simulink model "ecualizador"  (R2017a)
settings: Solver=FixedStepDiscrete  StartTime=0.0  StopTime=Inf  RelTol=1e-3  EnableMultiTasking=on
libraries: dsparch4 x7, dspsrcs4 x3, dspvision x1
settings Model: Creator=The MathWorks, Inc.  LastModifiedBy=hmartiney
settings DataIOCC: LimitDataPoints=on  SaveFormat=Array
settings OptimizationCC: LifeSpan=inf
settings DebuggingCC: SolverPrmCheckMsg=warning  AllowSymbolicDim=off  SFUnexpectedBacktrackingDiag=warning  SFNoUnconditionalDefaultTransitionDiag=warning  SFExecutionAtInitializationDiag=none
settings HardwareCC: ProdBitPerPointer=32  ProdBitPerSizeT=32  ProdBitPerPtrDiffT=32  ProdLargestAtomicFloat=None  ProdIntDivRoundTo=Undefined  ProdEndianess=Unspecified  ProdWordSize=32  ProdHWDeviceType=32-bit Generic
settings ModelReferenceCC: PropagateSignalLabelsOutOfModel=off
settings GRTTargetCC: TargetLangStandard=C89/C90 (ANSI)  GeneratePreprocessorConditionals=Disable all
settings ConfigComp: CovMetricSettings=dw  CovHtmlReporting=on  CovSaveCumulativeToWorkspaceVar=on  CovSaveSingleToWorkspaceVar=on  CovExternalEMLEnable=off  CovSFcnEnable=off

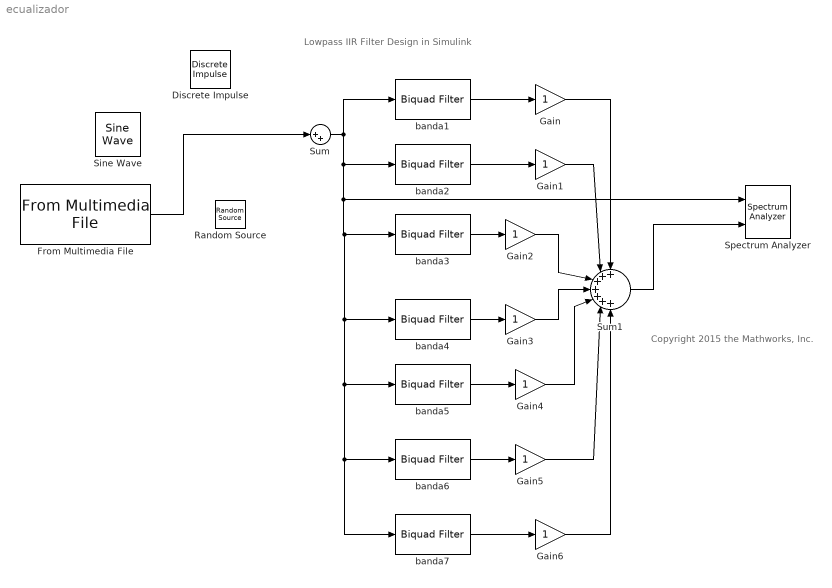
== system ecualizador ==
  note: Copyright 2015 the Mathworks, Inc.
  note: Lowpass IIR Filter Design in Simulink
  Discrete Impulse : dspsrcs4/Discrete  Impulse  Delay=0  SampleTime=1  FrameSample=1  OutputFrames=off  dataType=double  isSigned=on  wordLen=16  udDataType=sfix(16)  fracBitsMode=Best precision  numFracBits=15  OutDataTypeStr=double  LastOutDataTypeStr=double
  From Multimedia File : dspvision/From Multimedia File  inputFilename=/Users/hmartiney/DSPEqualizerProject/1-01 Out My Head (www.hiphopeasy.com).mp3  loop=on  numPlays=inf  outputStreams=Audio only  videoDataType=single  audioDataType=double  inheritSampleTime=on  userDefinedSampleTime=1/30  noAudioOutput=off  isIntensityVideo=off  fourcc=RGB  colorVideoFormat=Separate color signals  outputEOF=off  dataOrg=Column-major  audioFrameSize=1024  computeAudioFrameSize=off  outSamplingMode=Sample based
      settings: SourceProductBaseCode=VP
  Gain{,1..6} (7 alike) : Gain
  Random Source : dspsrcs4/Random Source  SrcType=Gaussian  NormMethod=Ziggurat  CltLength=12  MinVal=0  MaxVal=1  MeanVal=0  VarVal=1e-5  RepMode=Specify seed  rawSeed=1  IsInherit=off  SampMode=Discrete  SampTime=1/44100  SampFrame=1024  DataType=Double  OutComplex=Real  OutputFrames=off
  Sine Wave : dspsrcs4/Sine Wave  Amplitude=1  Frequency=100  Phase=0  SampleMode=Discrete  OutComplex=Real  CompMethod=Trigonometric fcn  TableSize=Speed  SampleTime=1/44100  SamplesPerFrame=1024  ResetState=Restart at time zero  OutputFrames=off  dataType=double  wordLen=16  udDataType=sfix(16)  fracBitsMode=Best precision  numFracBits=15  OutDataTypeStr=double  LastOutDataTypeStr=double
  Spectrum Analyzer : SpectrumAnalyzer  NumInputPorts=2
  Sum : Sum  Inputs=|++
  Sum1 : Sum  Inputs=+++++++
  banda1 : dsparch4/Biquad Filter  Tag=BlockMethodSubSystem  IIRFiltStruct=Direct form II  CoeffSource=Specify via dialog  BiQuadCoeffs=[0.00018458300227112165 -0.00036906768600448764 0.000184583002271121677 1 -1.99947854026079197 0.999478638598126135;0.00057538077100641725 -0.00115066319336694063 0.000575380771006417358 1 -1.99987759640344676 0.9998776947219844;2.27833399804225939e-05 -4.54683566244835644e-05 2.27833399804225905e-05 1 -1.99938484320312182 0.999384941551767825;1.00011892756945397 -2 1.00011892756945375 1 -1.99965158871292981 0.999651687036266057]  a0Flag=Warning  IC=0  ICnum=0  ICden=0  InputProcessing=Columns as channels (frame based)  denAccumFracLength=30  denProdOutputFracLength=30  secondMemoryFracLength=15  roundingMode=Floor  overflowMode=off  ScaleValues=[9.83373342755555768e-08;1;1;1;4204.23962093165483]  optimizeScaleValues=on  ScaleValueMode=Specify via input port (g)  scaleValueFracLength=14  FilterSource=Specify via dialog  FilterObject=BQF
      settings: SourceProductName=DSP System Toolbox
  banda2 : dsparch4/Biquad Filter  Tag=BlockMethodSubSystem  IIRFiltStruct=Direct form II  CoeffSource=Specify via dialog  BiQuadCoeffs=[0.192137146734570385 -0.384037148070295542 0.192137146734570385 1 -1.99777092121242461 0.999494811108345704;0.0756226935951563178 -0.151052150183008216 0.075622693595156304 1 -1.99765102526638483 0.999479693593270158;0.0721798852515740386 -0.144305358912791171 0.0721798852515740663 1 -1.99700920616910249 0.998762370564236002;1.00209566000222439 -1.99999999999999978 1.00209566000222439 1 -1.99695025262914783 0.99874706897447596]  a0Flag=Warning  IC=0  ICnum=0  ICden=0  InputProcessing=Columns as channels (frame based)  denAccumFracLength=30  denProdOutputFracLength=30  secondMemoryFracLength=15  roundingMode=Floor  overflowMode=off  ScaleValues=[2.28356136424982117e-05;1;1;1;416.112600169732445]  optimizeScaleValues=on  ScaleValueMode=Specify via input port (g)  scaleValueFracLength=14  FilterSource=Specify via dialog  FilterObject=BQF
      settings: SourceProductName=DSP System Toolbox
  banda3 : dsparch4/Biquad Filter  Tag=BlockMethodSubSystem  IIRFiltStruct=Direct form II  CoeffSource=Specify via dialog  BiQuadCoeffs=[0.180047662333926051 -0.359206709516307732 0.180047662333926051 1 -1.99209861256290632 0.998989800786029836;0.0769354203253417995 -0.153084985509638283 0.0769354203253417857 1 -1.99164983255421402 0.998959632781060591;0.0779338535689544365 -0.155632796369424647 0.0779338535689544504 1 -1.99052052081238928 0.997526120123505167;1.00842325818531764 -1.99999999999999978 1.00842325818531742 1 -1.99031570422060278 0.997495607254762273]  a0Flag=Warning  IC=0  ICnum=0  ICden=0  InputProcessing=Columns as channels (frame based)  denAccumFracLength=30  denProdOutputFracLength=30  secondMemoryFracLength=15  roundingMode=Floor  overflowMode=off  ScaleValues=[8.80922845753380219e-05;1;1;1;104.07738543556286]  optimizeScaleValues=on  ScaleValueMode=Specify via input port (g)  scaleValueFracLength=14  FilterSource=Specify via dialog  FilterObject=BQF
      settings: SourceProductName=DSP System Toolbox
  banda4 : dsparch4/Biquad Filter  Tag=BlockMethodSubSystem  IIRFiltStruct=Direct form II  CoeffSource=Specify via dialog  BiQuadCoeffs=[0.505126157663120412 -1.00884123578502005 0.505126157663120301 1 -1.97359600824949655 0.990179649727085387;0.228063336916342174 -0.455988024253138113 0.228063336916342174 1 -1.96419171567385797 0.988200848679448907;0.043263411634023731 -0.0804544298590833262 0.043263411634023724 1 -1.95659726538862322 0.974928349386933069;1.40151684739692706 -2 1.40151684739692772 1 -1.95154878665663123 0.972940389926792215]  a0Flag=Warning  IC=0  ICnum=0  ICden=0  InputProcessing=Columns as channels (frame based)  denAccumFracLength=30  denProdOutputFracLength=30  secondMemoryFracLength=15  roundingMode=Floor  overflowMode=off  ScaleValues=[0.00126472660708423995;1;1;1;1.29397976421985406]  optimizeScaleValues=on  ScaleValueMode=Specify via input port (g)  scaleValueFracLength=14  FilterSource=Specify via dialog  FilterObject=BQF
      settings: SourceProductName=DSP System Toolbox
  banda5 : dsparch4/Biquad Filter  Tag=BlockMethodSubSystem  IIRFiltStruct=Direct form II  CoeffSource=Specify via dialog  BiQuadCoeffs=[0.858450663015004944 -1.71124664016059302 0.858450663015004833 1 -1.88259186350801455 0.963726957045161425;0.366655713213130452 -0.732854894355177033 0.366655713213130452 1 -1.80172790029073271 0.95134369490768167;0.0370246853101634174 -0.0240418540911722309 0.0370246853101634105 1 -1.81144976937368929 0.90567029278450073;0.358370548386829246 0.329380028636398259 0.358370548386829191 1 -1.77197485426835666 0.8935808405627228]  a0Flag=Warning  IC=0  ICnum=0  ICden=0  InputProcessing=Columns as channels (frame based)  denAccumFracLength=30  denProdOutputFracLength=30  secondMemoryFracLength=15  roundingMode=Floor  overflowMode=off  ScaleValues=[0.0102988709524170011;1;1;1;1]  optimizeScaleValues=on  ScaleValueMode=Specify via input port (g)  scaleValueFracLength=14  FilterSource=Specify via dialog  FilterObject=BQF
      settings: SourceProductName=DSP System Toolbox
  banda6 : dsparch4/Biquad Filter  Tag=BlockMethodSubSystem  IIRFiltStruct=Direct form II  CoeffSource=Specify via dialog  BiQuadCoeffs=[0.701144681983514317 -1.37583661164337467 0.701144681983514206 1 -1.4336771181893313 0.90925136869741241;0.355690266735428362 -0.708870197882475406 0.355690266735428418 1 -1.04172055397109387 0.886777477869309272;0.0873388487512413436 0.108902451275647447 0.0873388487512413436 1 -1.24875342125452082 0.776277989253797429;0.328251331068859398 0.602303407299513149 0.328251331068859398 1 -1.08663904861009097 0.755759783368092575]  a0Flag=Warning  IC=0  ICnum=0  ICden=0  InputProcessing=Columns as channels (frame based)  denAccumFracLength=30  denProdOutputFracLength=30  secondMemoryFracLength=15  roundingMode=Floor  overflowMode=off  ScaleValues=[0.0598431123171891954;1;1;1;1]  optimizeScaleValues=on  ScaleValueMode=Specify via input port (g)  scaleValueFracLength=14  FilterSource=Specify via dialog  FilterObject=BQF
      settings: SourceProductName=DSP System Toolbox
  banda7 : dsparch4/Biquad Filter  Tag=BlockMethodSubSystem  IIRFiltStruct=Direct form II  CoeffSource=Specify via dialog  BiQuadCoeffs=[0.11385500982914995 -0.176173309938275569 0.11385500982915002 1 0.407591725889754009 0.141044415828899677;0.478369170533914811 -0.412302142752011491 0.478369170533915034 1 0.702865577600154445 0.720400056292610391;0.196866857971742748 -0.381535209742158932 0.196866857971742776 1 0.346926018697040539 0.0410803694216345799;0.445485009089283068 -0.494881474963274781 0.445485009089283068 1 0.525223218259760927 0.352581749330066863]  a0Flag=Warning  IC=0  ICnum=0  ICden=0  InputProcessing=Columns as channels (frame based)  denAccumFracLength=30  denProdOutputFracLength=30  secondMemoryFracLength=15  roundingMode=Floor  overflowMode=off  ScaleValues=[0.721489058510264014;1;1;1;1]  optimizeScaleValues=on  ScaleValueMode=Specify via input port (g)  scaleValueFracLength=14  FilterSource=Specify via dialog  FilterObject=BQF
      settings: SourceProductName=DSP System Toolbox
  wires:
  Sum1/1 -> Spectrum Analyzer/2
  Sum/1 -> banda1/1, banda2/1, Spectrum Analyzer/1, banda7/1, banda6/1, banda5/1, banda4/1, banda3/1
  banda2/1 -> Gain1/1
  banda1/1 -> Gain/1
  banda3/1 -> Gain2/1
  banda4/1 -> Gain3/1
  banda5/1 -> Gain4/1
  banda6/1 -> Gain5/1
  banda7/1 -> Gain6/1
  Gain/1 -> Sum1/1
  Gain1/1 -> Sum1/2
  Gain2/1 -> Sum1/3
  Gain3/1 -> Sum1/4
  Gain4/1 -> Sum1/5
  Gain5/1 -> Sum1/6
  Gain6/1 -> Sum1/7
  From Multimedia File/1 -> Sum/1
